simulink model "q3_2_1"  (R2022a)
settings: Solver=FixedStepAuto  StartTime=0.0  StopTime=20  FixedStep=5e-3  RelTol=1e-3
settings Model: Creator=armooga4  LastModifiedBy=user
settings SolverCC: AlgebraicLoopSolver=TrustRegion
settings DataIOCC: ReturnWorkspaceOutputs=off
settings DebuggingCC: UnconnectedInputMsg=warning  UnconnectedOutputMsg=warning  UnconnectedLineMsg=warning  SFMachineParentedDataDiag=warning  ArithmeticOperatorsInVariantConditions=warning
settings SFSimCC: SimUseLocalCustomCode=off  CustomCodeUndefinedFunction=UseInterfaceOnly
settings RTWCC: RTWUseLocalCustomCode=off

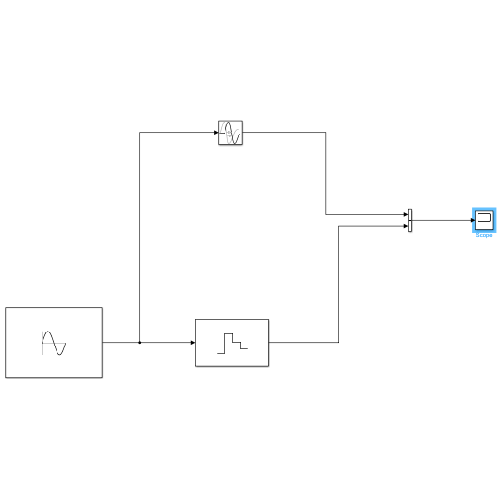
[thumbnail: Simulink's stored preview of the top-level diagram]
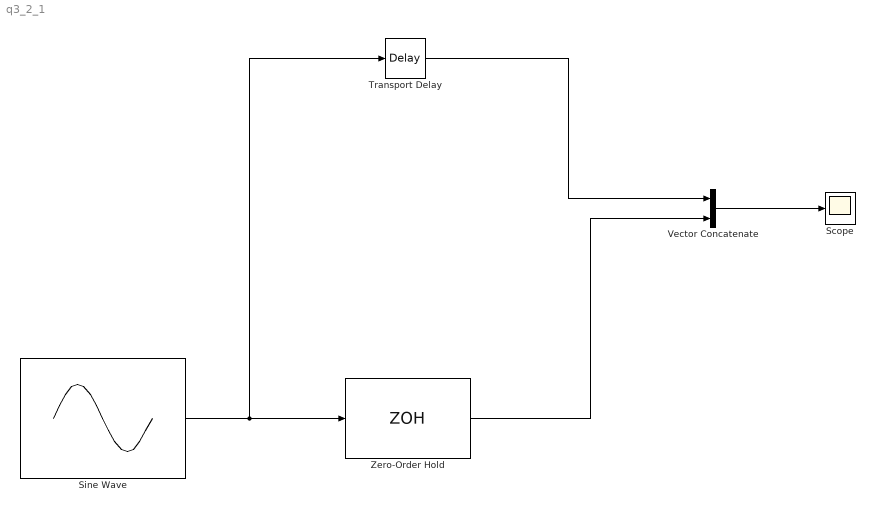
== system q3_2_1 ==
  Scope : Scope
  Sine Wave : Sin  Frequency=0.5  SampleTime=0
  Transport Delay : TransportDelay  DelayTime=0.5
  Vector Concatenate : Concatenate
  Zero-Order Hold : ZeroOrderHold
  wires:
  Sine Wave/1 -> Transport Delay/1, Zero-Order Hold/1
  Transport Delay/1 -> Vector Concatenate/1
  Zero-Order Hold/1 -> Vector Concatenate/2
  Vector Concatenate/1 -> Scope/1
